simulink model "Valve"  (R2024b)
settings: Solver=VariableStepAuto  StartTime=0.0  StopTime=10.0  RelTol=1e-3
settings Model: Creator=Steve  LastModifiedBy=Steve
settings ConfigComp: CovBoundaryAbsTol=1.0e-5

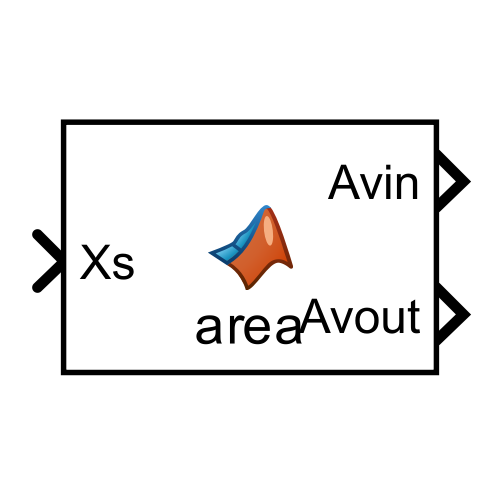
[thumbnail: Simulink's stored preview of the top-level diagram]
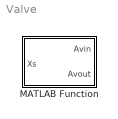
== system Valve ==
  MATLAB Function : MATLAB Function  TreatAsAtomicUnit=on

== matlab function Valve/MATLAB Function ==
  data: Xs input; Avin output; Avout output
function [Avin,Avout]= area(Xs)
nh = 4;
Pw = 0.0024;
Rh = 0.0019;
ph1 = 2*Rh^2*atan(sqrt((Rh-Pw+Xs)/(Rh+Pw-Xs)))-(Pw-Xs)*sqrt(Rh^2 - (Pw - Xs)^2);
ph2 = 2*Rh^2*atan(sqrt((Rh-Pw+abs(Xs))/(Rh+Pw-abs(Xs))))-(Pw-abs(Xs))*sqrt(Rh^2 - (Pw - abs(Xs))^2);
if Xs<=Pw-Rh
    Avin = 0;
elseif (Pw-Rh<Xs)&&(Xs<Pw+Rh)
    Avin = nh*ph1;
elseif Xs >= Pw+Rh
    Avin = pi*nh*Rh^2;
end

if Xs<=Pw-Rh
    Avout = pi*nh*Rh^2;
elseif (-Pw-Rh<Xs)&&(Xs<-Pw+Rh)
    Avout = nh*ph2;
elseif Xs >=-Pw+Rh
    Avout = 0;
end

end
